simulink model "EZE557StEnCtrl"  (R2018b)
settings: Solver=FixedStepDiscrete  StartTime=0.0  StopTime=10.0  FixedStep=0.01  RelTol=1e-3
undefined symbols (not defined in the file or in its folder): data, KeSMSw4SSecRwLtStLgrstOtwdInwdClosePos1_Val, KeSMSw4SSecRwLtStLgrstUpwdDnwdClosePos1_Val, KeSMSw4SSecRwLtStLgrstUpwdDnwdClosePos2_Val, PassStBkReclnEn_Clear, PassStBkReclnEn_Set, PassStFwdBkwdEn_Clear, PassStFwdBkwdEn_Set, SecRwLtStBkReclnEn_Clear, SecRwLtStBkReclnEn_Set, SecRwLtStFwdBkwdEn_Clear, SecRwLtStFwdBkwdEn_Set, SecRwLtStLgrstInwdOtwdEn_Clear, SecRwLtStLgrstInwdOtwdEn_Set, SecRwLtStLgrstUpwdDnwdEn_Clear, SecRwLtStLgrstUpwdDnwdEn_Set, SecRwRtStBkReclnEn_Clear, SecRwRtStBkReclnEn_Set, SecRwRtStFwdBkwdEn_Clear, SecRwRtStFwdBkwdEn_Set, SecRwRtStLgrstInwdOtwdEn_Clear, SecRwRtStLgrstInwdOtwdEn_Set, SecRwRtStLgrstUpwdDnwdEn_Clear, SecRwRtStLgrstUpwdDnwdEn_Set, ThdRwLtStBkReclnEn_Clear, ThdRwLtStBkReclnEn_Set, ThdRwLtStCshnFldEn_Clear, ThdRwLtStCshnFldEn_Set, ThdRwLtStFwdBkwdEn_Clear, ThdRwLtStFwdBkwdEn_Set, ThdRwRtStBkReclnEn_Clear, ThdRwRtStBkReclnEn_Set, ThdRwRtStCshnFldEn_Clear, ThdRwRtStCshnFldEn_Set, ThdRwRtStFwdBkwdEn_Clear, ThdRwRtStFwdBkwdEn_Set, ZeroLEn_Clear, ZeroLEn_Set, ZeroREn_Clear, ZeroREn_Set
libraries: simulink x1
(part 1 of 2)
settings Model: Creator=sn2xws  LastModifiedBy=sn55gm
settings Model: ModifiedHistory=|
  | 2024.5.7 V1.0.0 557 eze模式
  | 2024.6.17 V1.1.0 座椅模式流程图V1.6
  | 2024.8.16 修复stage1会退出的问题
  | 2024.8.17 二排靠背电机目标位置异常问题修复
  | 2024.8.29 V3.0.3 V2.4流程，如果二排靠背小于目标位置，第一阶段不动二排靠背
  | 2024.9.25 V3.0.4 二排靠背reset条件改为只在第一阶段完成后reset一次
  | 2024.11.12 V3.0.5 第一阶段二排靠背到位置的flag替换
settings DataIOCC: SaveFormat=StructureWithTime
settings OptimizationCC: DefaultParameterBehavior=Inlined  EnhancedBackFolding=on  PassReuseOutputArgsAs=Individual arguments  ZeroExternalMemoryAtStartup=off  ZeroInternalMemoryAtStartup=off  OptimizeBlockOrder=speed  DifferentSizesBufferReuse=on  OptimizationCustomize=off
settings DebuggingCC: ParameterTunabilityLossMsg=error
settings SFSimCC: MATLABDynamicMemAlloc=off
settings RTWCC: SystemTargetFile=autosar.tlc  GenCodeOnly=on  TemplateMakefile=ert_default_tmf  Description=AUTOSAR  GenerateReport=on  IncludeHyperlinkInReport=on  LaunchReport=on  GenerateTraceInfo=on  GenerateTraceReport=on  GenerateTraceReportSl=on  GenerateTraceReportSf=on  GenerateTraceReportEml=on
settings CodeAppCC: ForceParamTrailComments=on  IgnoreCustomStorageClasses=off  OperatorAnnotations=on  SimulinkDataObjDesc=on  SFDataObjDesc=on  InsertBlockDesc=on
settings STFCustomTargetCC: TargetLangStandard=C99 (ISO)  MultiwordLength=256  ParMdlRefBuildCompliant=on  CompOptLevelCompliant=on  IncludeMdlTerminateFcn=off  CombineOutputUpdateFcns=on  SuppressErrorStatus=on  ERTCustomFileBanners=on  SupportNonFinite=off  SupportComplex=off  SupportContinuousTime=off  SupportNonInlinedSFcns=off  RemoveResetFunc=on  MATLABClassNameForMDSCustomization=Simulink.SoftwareTarget.ERTCustomization  AutosarCompliant=on  UseToolchainInfoCompliant=on  LookupTableObjectStructAxisOrder=2,1,3,4,...  LUTObjectStructOrderEvenSpacing=Size,Table,Breakpoints  SystemTargetFile=autosar.tlc
settings ERTTargetCC: TargetLangStandard=C99 (ISO)  ConcurrentExecutionCompliant=off  IncludeMdlTerminateFcn=off  SuppressErrorStatus=on  SupportNonFinite=off  SupportComplex=off  ModelStepFunctionPrototypeControlCompliant=off  CPPClassGenCompliant=off  AutosarCompliant=on  LookupTableObjectStructAxisOrder=2,1,3,4,...  LUTObjectStructOrderEvenSpacing=Size,Table,Breakpoints  InlinedParameterPlacement=NonHierarchical  ERTCustomFileTemplate=example_file_process.tlc  ERTFilePackagingFormat=Compact  BooleanTrueId=TRUE  BooleanFalseId=FALSE

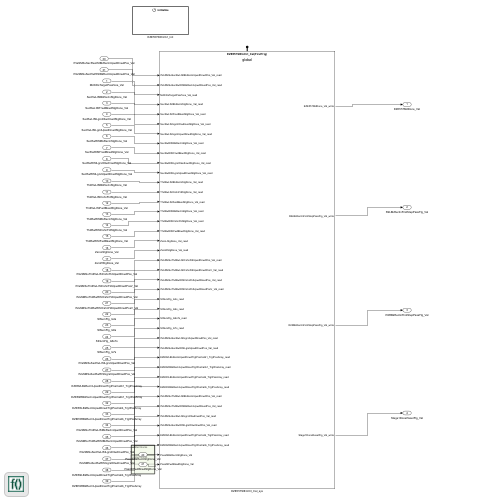
[thumbnail: Simulink's stored preview of the top-level diagram]
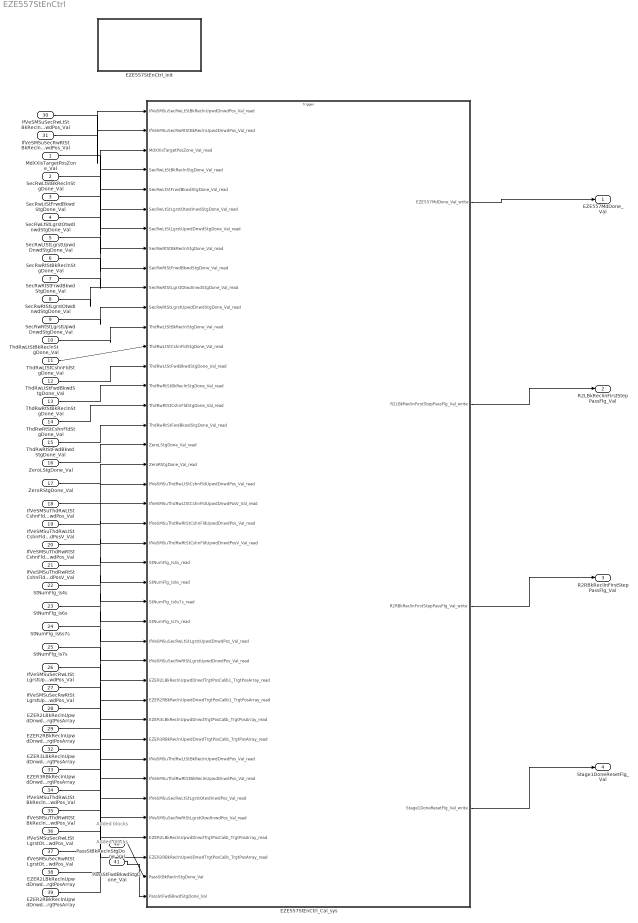
== system EZE557StEnCtrl ==
  note: Added blocks
  note: Added blocks
  MdXXIsTargetPosZone_Val : Inport  OutDataTypeStr=uint32  PortDimensions=1
  SecRwLtStBkReclnStgDone_Val : Inport  Port=2  OutDataTypeStr=boolean  PortDimensions=1
  SecRwLtStFrwdBkwdStgDone_Val : Inport  Port=3  OutDataTypeStr=boolean  PortDimensions=1
  SecRwLtStLgrstOtwdInwdStgDone_Val : Inport  Port=4  OutDataTypeStr=boolean  PortDimensions=1
  SecRwLtStLgrstUpwdDnwdStgDone_Val : Inport  Port=5  OutDataTypeStr=boolean  PortDimensions=1
  SecRwRtStBkReclnStgDone_Val : Inport  Port=6  OutDataTypeStr=boolean  PortDimensions=1
  SecRwRtStFrwdBkwdStgDone_Val : Inport  Port=7  OutDataTypeStr=boolean  PortDimensions=1
  SecRwRtStLgrstOtwdInwdStgDone_Val : Inport  Port=8  OutDataTypeStr=boolean  PortDimensions=1
  SecRwRtStLgrstUpwdDnwdStgDone_Val : Inport  Port=9  OutDataTypeStr=boolean  PortDimensions=1
  ThdRwLtStBkReclnStgDone_Val : Inport  Port=10  OutDataTypeStr=boolean  PortDimensions=1
  ThdRwLtStCshnFldStgDone_Val : Inport  Port=11  OutDataTypeStr=boolean  PortDimensions=1
  ThdRwLtStFwdBkwdStgDone_Val : Inport  Port=12  OutDataTypeStr=boolean  PortDimensions=1
  ThdRwRtStBkReclnStgDone_Val : Inport  Port=13  OutDataTypeStr=boolean  PortDimensions=1
  ThdRwRtStCshnFldStgDone_Val : Inport  Port=14  OutDataTypeStr=boolean  PortDimensions=1
  ThdRwRtStFwdBkwdStgDone_Val : Inport  Port=15  OutDataTypeStr=boolean  PortDimensions=1
  ZeroLStgDone_Val : Inport  Port=16  OutDataTypeStr=boolean  PortDimensions=1
  ZeroRStgDone_Val : Inport  Port=17  OutDataTypeStr=boolean  PortDimensions=1
  IfVeSMSuThdRwLtStCshnFldUpwdDnwdPos_Val : Inport  Port=18  OutDataTypeStr=uint16  PortDimensions=1
  IfVeSMSuThdRwLtStCshnFldUpwdDnwdPosV_Val : Inport  Port=19  OutDataTypeStr=boolean  PortDimensions=1
  IfVeSMSuThdRwRtStCshnFldUpwdDnwdPos_Val : Inport  Port=20  OutDataTypeStr=uint16  PortDimensions=1
  IfVeSMSuThdRwRtStCshnFldUpwdDnwdPosV_Val : Inport  Port=21  OutDataTypeStr=boolean  PortDimensions=1
  StNumFlg_Is4s : Inport  Port=22  OutDataTypeStr=boolean  PortDimensions=1
  StNumFlg_Is6s : Inport  Port=23  OutDataTypeStr=boolean  PortDimensions=1
  StNumFlg_Is6s7s : Inport  Port=24  OutDataTypeStr=boolean  PortDimensions=1
  StNumFlg_Is7s : Inport  Port=25  OutDataTypeStr=boolean  PortDimensions=1
  IfVeSMSuSecRwLtStLgrstUpwdDnwdPos_Val : Inport  Port=26  OutDataTypeStr=uint16  PortDimensions=1
  IfVeSMSuSecRwRtStLgrstUpwdDnwdPos_Val : Inport  Port=27  OutDataTypeStr=uint16  PortDimensions=1
  EZER2LBkReclnUpwdDnwdTrgtPosCalib1_TrgtPosArray : Inport  Description=|  Port=28  OutDataTypeStr=uint16  PortDimensions=3
      | 0:Pos
      | 1:Max
      | 2:Min
  EZER2RBkReclnUpwdDnwdTrgtPosCalib1_TrgtPosArray : Inport  Description=|  Port=29  OutDataTypeStr=uint16  PortDimensions=3
      | 0:Pos
      | 1:Max
      | 2:Min
  IfVeSMSuSecRwLtStBkReclnUpwdDnwdPos_Val : Inport  Port=30  OutDataTypeStr=uint16  PortDimensions=1
  IfVeSMSuSecRwRtStBkReclnUpwdDnwdPos_Val : Inport  Port=31  OutDataTypeStr=uint16  PortDimensions=1
  EZER3LBkReclnUpwdDnwdTrgtPosCalib_TrgtPosArray : Inport  Description=|  Port=32  OutDataTypeStr=uint16  PortDimensions=3
      | 0:Pos
      | 1:Max
      | 2:Min
  EZER3RBkReclnUpwdDnwdTrgtPosCalib_TrgtPosArray : Inport  Description=|  Port=33  OutDataTypeStr=uint16  PortDimensions=3
      | 0:Pos
      | 1:Max
      | 2:Min
  IfVeSMSuThdRwLtStBkReclnUpwdDnwdPos_Val : Inport  Port=34  OutDataTypeStr=uint16  PortDimensions=1
  IfVeSMSuThdRwRtStBkReclnUpwdDnwdPos_Val : Inport  Port=35  OutDataTypeStr=uint16  PortDimensions=1
  IfVeSMSuSecRwLtStLgrstOtwdInwdPos_Val : Inport  Port=36  OutDataTypeStr=uint16  PortDimensions=1
  IfVeSMSuSecRwRtStLgrstOtwdInwdPos_Val : Inport  Port=37  OutDataTypeStr=uint16  PortDimensions=1
  EZER2LBkReclnUpwdDnwdTrgtPosCalib_TrgtPosArray : Inport  Description=|  Port=38  OutDataTypeStr=uint16  PortDimensions=3
      | 0:Pos
      | 1:Max
      | 2:Min
  EZER2RBkReclnUpwdDnwdTrgtPosCalib_TrgtPosArray : Inport  Description=|  Port=39  OutDataTypeStr=uint16  PortDimensions=3
      | 0:Pos
      | 1:Max
      | 2:Min
  PassStBkReclnStgDone_Val : Inport  Port=40  OutDataTypeStr=boolean  PortDimensions=1
  PassStFwdBkwdStgDone_Val : Inport  Port=41  OutDataTypeStr=boolean  PortDimensions=1
  EZE557StEnCtrl_Cal_sys : Subsystem
  EZE557StEnCtrl_Init : Subsystem
  EZE557MdDone_Val : Outport  OutDataTypeStr=uint8  PortDimensions=1  VectorParamsAs1DForOutWhenUnconnected=off
  R2LBkReclinFirstStepPassFlg_Val : Outport  Port=2  OutDataTypeStr=boolean  PortDimensions=1  VectorParamsAs1DForOutWhenUnconnected=off
  R2RBkReclinFirstStepPassFlg_Val : Outport  Port=3  OutDataTypeStr=boolean  PortDimensions=1  VectorParamsAs1DForOutWhenUnconnected=off
  Stage1DoneResetFlg_Val : Outport  Port=4  OutDataTypeStr=boolean  PortDimensions=1  VectorParamsAs1DForOutWhenUnconnected=off
  wires:
  MdXXIsTargetPosZone_Val/1 -> EZE557StEnCtrl_Cal_sys/3(MdXXIsTargetPosZone_Val_read)
  SecRwLtStBkReclnStgDone_Val/1 -> EZE557StEnCtrl_Cal_sys/4(SecRwLtStBkReclnStgDone_Val_read)
  SecRwLtStFrwdBkwdStgDone_Val/1 -> EZE557StEnCtrl_Cal_sys/5(SecRwLtStFrwdBkwdStgDone_Val_read)
  SecRwLtStLgrstOtwdInwdStgDone_Val/1 -> EZE557StEnCtrl_Cal_sys/6(SecRwLtStLgrstOtwdInwdStgDone_Val_read)
  SecRwLtStLgrstUpwdDnwdStgDone_Val/1 -> EZE557StEnCtrl_Cal_sys/7(SecRwLtStLgrstUpwdDnwdStgDone_Val_read)
  SecRwRtStBkReclnStgDone_Val/1 -> EZE557StEnCtrl_Cal_sys/8(SecRwRtStBkReclnStgDone_Val_read)
  SecRwRtStFrwdBkwdStgDone_Val/1 -> EZE557StEnCtrl_Cal_sys/9(SecRwRtStFrwdBkwdStgDone_Val_read)
  SecRwRtStLgrstOtwdInwdStgDone_Val/1 -> EZE557StEnCtrl_Cal_sys/10(SecRwRtStLgrstOtwdInwdStgDone_Val_read)
  SecRwRtStLgrstUpwdDnwdStgDone_Val/1 -> EZE557StEnCtrl_Cal_sys/11(SecRwRtStLgrstUpwdDnwdStgDone_Val_read)
  ThdRwLtStBkReclnStgDone_Val/1 -> EZE557StEnCtrl_Cal_sys/12(ThdRwLtStBkReclnStgDone_Val_read)
  ThdRwLtStCshnFldStgDone_Val/1 -> EZE557StEnCtrl_Cal_sys/13(ThdRwLtStCshnFldStgDone_Val_read)
  ThdRwLtStFwdBkwdStgDone_Val/1 -> EZE557StEnCtrl_Cal_sys/14(ThdRwLtStFwdBkwdStgDone_Val_read)
  ThdRwRtStBkReclnStgDone_Val/1 -> EZE557StEnCtrl_Cal_sys/15(ThdRwRtStBkReclnStgDone_Val_read)
  ThdRwRtStCshnFldStgDone_Val/1 -> EZE557StEnCtrl_Cal_sys/16(ThdRwRtStCshnFldStgDone_Val_read)
  ThdRwRtStFwdBkwdStgDone_Val/1 -> EZE557StEnCtrl_Cal_sys/17(ThdRwRtStFwdBkwdStgDone_Val_read)
  ZeroLStgDone_Val/1 -> EZE557StEnCtrl_Cal_sys/18(ZeroLStgDone_Val_read)
  ZeroRStgDone_Val/1 -> EZE557StEnCtrl_Cal_sys/19(ZeroRStgDone_Val_read)
  EZE557StEnCtrl_Cal_sys/1(EZE557MdDone_Val_write) -> EZE557MdDone_Val/1
  IfVeSMSuThdRwLtStCshnFldUpwdDnwdPos_Val/1 -> EZE557StEnCtrl_Cal_sys/20(IfVeSMSuThdRwLtStCshnFldUpwdDnwdPos_Val_read)
  IfVeSMSuThdRwLtStCshnFldUpwdDnwdPosV_Val/1 -> EZE557StEnCtrl_Cal_sys/21(IfVeSMSuThdRwLtStCshnFldUpwdDnwdPosV_Val_read)
  IfVeSMSuThdRwRtStCshnFldUpwdDnwdPos_Val/1 -> EZE557StEnCtrl_Cal_sys/22(IfVeSMSuThdRwRtStCshnFldUpwdDnwdPos_Val_read)
  IfVeSMSuThdRwRtStCshnFldUpwdDnwdPosV_Val/1 -> EZE557StEnCtrl_Cal_sys/23(IfVeSMSuThdRwRtStCshnFldUpwdDnwdPosV_Val_read)
  StNumFlg_Is4s/1 -> EZE557StEnCtrl_Cal_sys/24(StNumFlg_Is4s_read)
  StNumFlg_Is6s/1 -> EZE557StEnCtrl_Cal_sys/25(StNumFlg_Is6s_read)
  StNumFlg_Is6s7s/1 -> EZE557StEnCtrl_Cal_sys/26(StNumFlg_Is6s7s_read)
  StNumFlg_Is7s/1 -> EZE557StEnCtrl_Cal_sys/27(StNumFlg_Is7s_read)
  IfVeSMSuSecRwLtStLgrstUpwdDnwdPos_Val/1 -> EZE557StEnCtrl_Cal_sys/28(IfVeSMSuSecRwLtStLgrstUpwdDnwdPos_Val_read)
  IfVeSMSuSecRwRtStLgrstUpwdDnwdPos_Val/1 -> EZE557StEnCtrl_Cal_sys/29(IfVeSMSuSecRwRtStLgrstUpwdDnwdPos_Val_read)
  EZER2LBkReclnUpwdDnwdTrgtPosCalib1_TrgtPosArray/1 -> EZE557StEnCtrl_Cal_sys/30(EZER2LBkReclnUpwdDnwdTrgtPosCalib1_TrgtPosArray_read)
  EZER2RBkReclnUpwdDnwdTrgtPosCalib1_TrgtPosArray/1 -> EZE557StEnCtrl_Cal_sys/31(EZER2RBkReclnUpwdDnwdTrgtPosCalib1_TrgtPosArray_read)
  IfVeSMSuSecRwLtStBkReclnUpwdDnwdPos_Val/1 -> EZE557StEnCtrl_Cal_sys/1(IfVeSMSuSecRwLtStBkReclnUpwdDnwdPos_Val_read)
  IfVeSMSuSecRwRtStBkReclnUpwdDnwdPos_Val/1 -> EZE557StEnCtrl_Cal_sys/2(IfVeSMSuSecRwRtStBkReclnUpwdDnwdPos_Val_read)
  EZE557StEnCtrl_Cal_sys/2(R2LBkReclinFirstStepPassFlg_Val_write) -> R2LBkReclinFirstStepPassFlg_Val/1
  EZE557StEnCtrl_Cal_sys/3(R2RBkReclinFirstStepPassFlg_Val_write) -> R2RBkReclinFirstStepPassFlg_Val/1
  EZER3LBkReclnUpwdDnwdTrgtPosCalib_TrgtPosArray/1 -> EZE557StEnCtrl_Cal_sys/32(EZER3LBkReclnUpwdDnwdTrgtPosCalib_TrgtPosArray_read)
  EZER3RBkReclnUpwdDnwdTrgtPosCalib_TrgtPosArray/1 -> EZE557StEnCtrl_Cal_sys/33(EZER3RBkReclnUpwdDnwdTrgtPosCalib_TrgtPosArray_read)
  IfVeSMSuThdRwLtStBkReclnUpwdDnwdPos_Val/1 -> EZE557StEnCtrl_Cal_sys/34(IfVeSMSuThdRwLtStBkReclnUpwdDnwdPos_Val_read)
  IfVeSMSuThdRwRtStBkReclnUpwdDnwdPos_Val/1 -> EZE557StEnCtrl_Cal_sys/35(IfVeSMSuThdRwRtStBkReclnUpwdDnwdPos_Val_read)
  EZE557StEnCtrl_Cal_sys/4(Stage1DoneResetFlg_Val_write) -> Stage1DoneResetFlg_Val/1
  IfVeSMSuSecRwLtStLgrstOtwdInwdPos_Val/1 -> EZE557StEnCtrl_Cal_sys/36(IfVeSMSuSecRwLtStLgrstOtwdInwdPos_Val_read)
  IfVeSMSuSecRwRtStLgrstOtwdInwdPos_Val/1 -> EZE557StEnCtrl_Cal_sys/37(IfVeSMSuSecRwRtStLgrstOtwdInwdPos_Val_read)
  EZER2LBkReclnUpwdDnwdTrgtPosCalib_TrgtPosArray/1 -> EZE557StEnCtrl_Cal_sys/38(EZER2LBkReclnUpwdDnwdTrgtPosCalib_TrgtPosArray_read)
  EZER2RBkReclnUpwdDnwdTrgtPosCalib_TrgtPosArray/1 -> EZE557StEnCtrl_Cal_sys/39(EZER2RBkReclnUpwdDnwdTrgtPosCalib_TrgtPosArray_read)
  PassStBkReclnStgDone_Val/1 -> EZE557StEnCtrl_Cal_sys/40(PassStBkReclnStgDone_Val)
  PassStFwdBkwdStgDone_Val/1 -> EZE557StEnCtrl_Cal_sys/41(PassStFwdBkwdStgDone_Val)

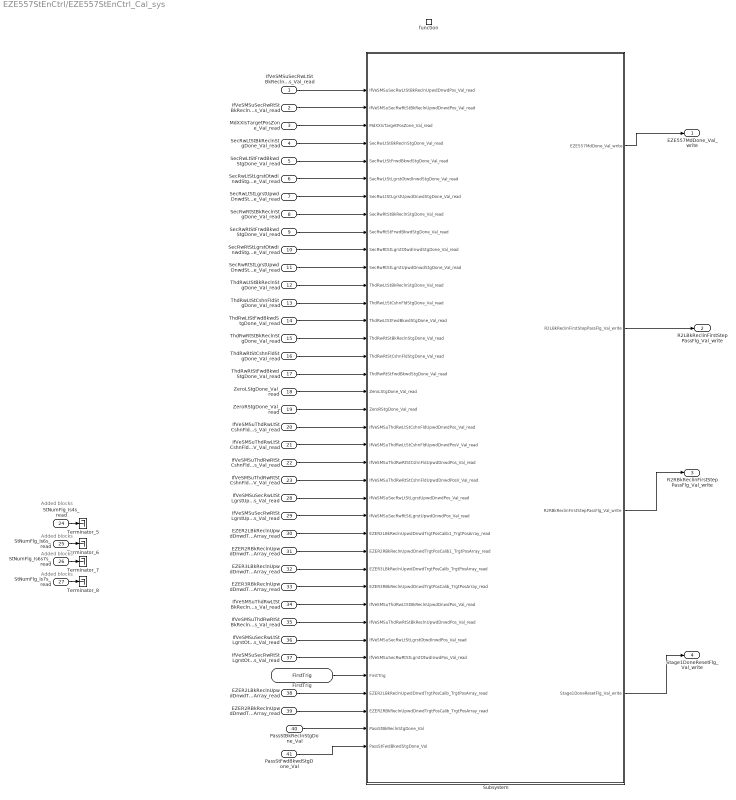
== system EZE557StEnCtrl/EZE557StEnCtrl_Cal_sys ==
  note: Added blocks
  note: Added blocks
  note: Added blocks
  note: Added blocks
  IfVeSMSuSecRwLtStBkReclnUpwdDnwdPos_Val_read : Inport
  IfVeSMSuSecRwRtStBkReclnUpwdDnwdPos_Val_read : Inport  Port=2
  MdXXIsTargetPosZone_Val_read : Inport  Port=3
  SecRwLtStBkReclnStgDone_Val_read : Inport  Port=4
  SecRwLtStFrwdBkwdStgDone_Val_read : Inport  Port=5
  SecRwLtStLgrstOtwdInwdStgDone_Val_read : Inport  Port=6
  SecRwLtStLgrstUpwdDnwdStgDone_Val_read : Inport  Port=7
  SecRwRtStBkReclnStgDone_Val_read : Inport  Port=8
  SecRwRtStFrwdBkwdStgDone_Val_read : Inport  Port=9
  SecRwRtStLgrstOtwdInwdStgDone_Val_read : Inport  Port=10
  SecRwRtStLgrstUpwdDnwdStgDone_Val_read : Inport  Port=11
  ThdRwLtStBkReclnStgDone_Val_read : Inport  Port=12
  ThdRwLtStCshnFldStgDone_Val_read : Inport  Port=13
  ThdRwLtStFwdBkwdStgDone_Val_read : Inport  Port=14
  ThdRwRtStBkReclnStgDone_Val_read : Inport  Port=15
  ThdRwRtStCshnFldStgDone_Val_read : Inport  Port=16
  ThdRwRtStFwdBkwdStgDone_Val_read : Inport  Port=17
  ZeroLStgDone_Val_read : Inport  Port=18
  ZeroRStgDone_Val_read : Inport  Port=19
  IfVeSMSuThdRwLtStCshnFldUpwdDnwdPos_Val_read : Inport  Port=20
  IfVeSMSuThdRwLtStCshnFldUpwdDnwdPosV_Val_read : Inport  Port=21
  IfVeSMSuThdRwRtStCshnFldUpwdDnwdPos_Val_read : Inport  Port=22
  IfVeSMSuThdRwRtStCshnFldUpwdDnwdPosV_Val_read : Inport  Port=23
  StNumFlg_Is4s_read : Inport  Port=24
  StNumFlg_Is6s_read : Inport  Port=25
  StNumFlg_Is6s7s_read : Inport  Port=26
  StNumFlg_Is7s_read : Inport  Port=27
  IfVeSMSuSecRwLtStLgrstUpwdDnwdPos_Val_read : Inport  Port=28
  IfVeSMSuSecRwRtStLgrstUpwdDnwdPos_Val_read : Inport  Port=29
  EZER2LBkReclnUpwdDnwdTrgtPosCalib1_TrgtPosArray_read : Inport  Port=30
  EZER2RBkReclnUpwdDnwdTrgtPosCalib1_TrgtPosArray_read : Inport  Port=31
  EZER3LBkReclnUpwdDnwdTrgtPosCalib_TrgtPosArray_read : Inport  Port=32
  EZER3RBkReclnUpwdDnwdTrgtPosCalib_TrgtPosArray_read : Inport  Port=33
  IfVeSMSuThdRwLtStBkReclnUpwdDnwdPos_Val_read : Inport  Port=34
  IfVeSMSuThdRwRtStBkReclnUpwdDnwdPos_Val_read : Inport  Port=35
  IfVeSMSuSecRwLtStLgrstOtwdInwdPos_Val_read : Inport  Port=36
  IfVeSMSuSecRwRtStLgrstOtwdInwdPos_Val_read : Inport  Port=37
  EZER2LBkReclnUpwdDnwdTrgtPosCalib_TrgtPosArray_read : Inport  Port=38
  EZER2RBkReclnUpwdDnwdTrgtPosCalib_TrgtPosArray_read : Inport  Port=39
  PassStBkReclnStgDone_Val : Inport  Port=40
  PassStFwdBkwdStgDone_Val : Inport  Port=41
  function : TriggerPort  TriggerType=function-call  IsSimulinkFunction=on  FunctionName=EZE557StEnCtrl_Cal  VariantControl=(inherit)
  Subsystem : Subsystem
  Terminator_{5..8} (4 alike) : Terminator
  FirstTrig : ArgIn  OutDataTypeStr=boolean  ArgumentName=FirstTrig
  EZE557MdDone_Val_write : Outport  VectorParamsAs1DForOutWhenUnconnected=off
      settings: EnsureOutportIsVirtual=on
  R2LBkReclinFirstStepPassFlg_Val_write : Outport  Port=2  VectorParamsAs1DForOutWhenUnconnected=off
      settings: EnsureOutportIsVirtual=on
  R2RBkReclinFirstStepPassFlg_Val_write : Outport  Port=3  VectorParamsAs1DForOutWhenUnconnected=off
      settings: EnsureOutportIsVirtual=on
  Stage1DoneResetFlg_Val_write : Outport  Port=4  VectorParamsAs1DForOutWhenUnconnected=off
      settings: EnsureOutportIsVirtual=on
  wires:
  MdXXIsTargetPosZone_Val_read/1 -> Subsystem/3(MdXXIsTargetPosZone_Val_read)
  SecRwLtStBkReclnStgDone_Val_read/1 -> Subsystem/4(SecRwLtStBkReclnStgDone_Val_read)
  SecRwLtStFrwdBkwdStgDone_Val_read/1 -> Subsystem/5(SecRwLtStFrwdBkwdStgDone_Val_read)
  SecRwLtStLgrstOtwdInwdStgDone_Val_read/1 -> Subsystem/6(SecRwLtStLgrstOtwdInwdStgDone_Val_read)
  SecRwLtStLgrstUpwdDnwdStgDone_Val_read/1 -> Subsystem/7(SecRwLtStLgrstUpwdDnwdStgDone_Val_read)
  SecRwRtStBkReclnStgDone_Val_read/1 -> Subsystem/8(SecRwRtStBkReclnStgDone_Val_read)
  SecRwRtStFrwdBkwdStgDone_Val_read/1 -> Subsystem/9(SecRwRtStFrwdBkwdStgDone_Val_read)
  SecRwRtStLgrstOtwdInwdStgDone_Val_read/1 -> Subsystem/10(SecRwRtStLgrstOtwdInwdStgDone_Val_read)
  SecRwRtStLgrstUpwdDnwdStgDone_Val_read/1 -> Subsystem/11(SecRwRtStLgrstUpwdDnwdStgDone_Val_read)
  ThdRwLtStBkReclnStgDone_Val_read/1 -> Subsystem/12(ThdRwLtStBkReclnStgDone_Val_read)
  ThdRwLtStCshnFldStgDone_Val_read/1 -> Subsystem/13(ThdRwLtStCshnFldStgDone_Val_read)
  ThdRwLtStFwdBkwdStgDone_Val_read/1 -> Subsystem/14(ThdRwLtStFwdBkwdStgDone_Val_read)
  ThdRwRtStBkReclnStgDone_Val_read/1 -> Subsystem/15(ThdRwRtStBkReclnStgDone_Val_read)
  ThdRwRtStCshnFldStgDone_Val_read/1 -> Subsystem/16(ThdRwRtStCshnFldStgDone_Val_read)
  ThdRwRtStFwdBkwdStgDone_Val_read/1 -> Subsystem/17(ThdRwRtStFwdBkwdStgDone_Val_read)
  ZeroLStgDone_Val_read/1 -> Subsystem/18(ZeroLStgDone_Val_read)
  ZeroRStgDone_Val_read/1 -> Subsystem/19(ZeroRStgDone_Val_read)
  Subsystem/1(EZE557MdDone_Val_write) -> EZE557MdDone_Val_write/1
  StNumFlg_Is4s_read/1 -> Terminator_5/1
  StNumFlg_Is6s_read/1 -> Terminator_6/1
  StNumFlg_Is6s7s_read/1 -> Terminator_7/1
  StNumFlg_Is7s_read/1 -> Terminator_8/1
  IfVeSMSuThdRwLtStCshnFldUpwdDnwdPos_Val_read/1 -> Subsystem/20(IfVeSMSuThdRwLtStCshnFldUpwdDnwdPos_Val_read)
  IfVeSMSuThdRwLtStCshnFldUpwdDnwdPosV_Val_read/1 -> Subsystem/21(IfVeSMSuThdRwLtStCshnFldUpwdDnwdPosV_Val_read)
  IfVeSMSuThdRwRtStCshnFldUpwdDnwdPos_Val_read/1 -> Subsystem/22(IfVeSMSuThdRwRtStCshnFldUpwdDnwdPos_Val_read)
  IfVeSMSuThdRwRtStCshnFldUpwdDnwdPosV_Val_read/1 -> Subsystem/23(IfVeSMSuThdRwRtStCshnFldUpwdDnwdPosV_Val_read)
  IfVeSMSuSecRwLtStLgrstUpwdDnwdPos_Val_read/1 -> Subsystem/24(IfVeSMSuSecRwLtStLgrstUpwdDnwdPos_Val_read)
  IfVeSMSuSecRwRtStLgrstUpwdDnwdPos_Val_read/1 -> Subsystem/25(IfVeSMSuSecRwRtStLgrstUpwdDnwdPos_Val_read)
  EZER2LBkReclnUpwdDnwdTrgtPosCalib1_TrgtPosArray_read/1 -> Subsystem/26(EZER2LBkReclnUpwdDnwdTrgtPosCalib1_TrgtPosArray_read)
  EZER2RBkReclnUpwdDnwdTrgtPosCalib1_TrgtPosArray_read/1 -> Subsystem/27(EZER2RBkReclnUpwdDnwdTrgtPosCalib1_TrgtPosArray_read)
  IfVeSMSuSecRwLtStBkReclnUpwdDnwdPos_Val_read/1 -> Subsystem/1(IfVeSMSuSecRwLtStBkReclnUpwdDnwdPos_Val_read)
  IfVeSMSuSecRwRtStBkReclnUpwdDnwdPos_Val_read/1 -> Subsystem/2(IfVeSMSuSecRwRtStBkReclnUpwdDnwdPos_Val_read)
  EZER3LBkReclnUpwdDnwdTrgtPosCalib_TrgtPosArray_read/1 -> Subsystem/28(EZER3LBkReclnUpwdDnwdTrgtPosCalib_TrgtPosArray_read)
  EZER3RBkReclnUpwdDnwdTrgtPosCalib_TrgtPosArray_read/1 -> Subsystem/29(EZER3RBkReclnUpwdDnwdTrgtPosCalib_TrgtPosArray_read)
  IfVeSMSuThdRwLtStBkReclnUpwdDnwdPos_Val_read/1 -> Subsystem/30(IfVeSMSuThdRwLtStBkReclnUpwdDnwdPos_Val_read)
  IfVeSMSuThdRwRtStBkReclnUpwdDnwdPos_Val_read/1 -> Subsystem/31(IfVeSMSuThdRwRtStBkReclnUpwdDnwdPos_Val_read)
  Subsystem/2(R2LBkReclinFirstStepPassFlg_Val_write) -> R2LBkReclinFirstStepPassFlg_Val_write/1
  Subsystem/3(R2RBkReclinFirstStepPassFlg_Val_write) -> R2RBkReclinFirstStepPassFlg_Val_write/1
  Subsystem/4(Stage1DoneResetFlg_Val_write) -> Stage1DoneResetFlg_Val_write/1
  IfVeSMSuSecRwLtStLgrstOtwdInwdPos_Val_read/1 -> Subsystem/32(IfVeSMSuSecRwLtStLgrstOtwdInwdPos_Val_read)
  IfVeSMSuSecRwRtStLgrstOtwdInwdPos_Val_read/1 -> Subsystem/33(IfVeSMSuSecRwRtStLgrstOtwdInwdPos_Val_read)
  FirstTrig/1 -> Subsystem/34(FirstTrig)
  EZER2LBkReclnUpwdDnwdTrgtPosCalib_TrgtPosArray_read/1 -> Subsystem/35(EZER2LBkReclnUpwdDnwdTrgtPosCalib_TrgtPosArray_read)
  EZER2RBkReclnUpwdDnwdTrgtPosCalib_TrgtPosArray_read/1 -> Subsystem/36(EZER2RBkReclnUpwdDnwdTrgtPosCalib_TrgtPosArray_read)
  PassStBkReclnStgDone_Val/1 -> Subsystem/37(PassStBkReclnStgDone_Val)
  PassStFwdBkwdStgDone_Val/1 -> Subsystem/38(PassStFwdBkwdStgDone_Val)

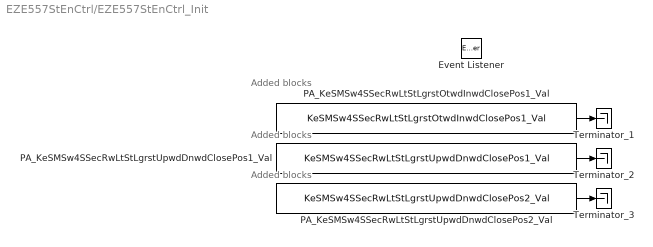
== system EZE557StEnCtrl/EZE557StEnCtrl_Init ==
  note: Added blocks
  note: Added blocks
  note: Added blocks
  Event Listener : EventListener  EventName=reset
  PA_KeSMSw4SSecRwLtStLgrstOtwdInwdClosePos1_Val : Constant  Value=KeSMSw4SSecRwLtStLgrstOtwdInwdClosePos1_Val
  PA_KeSMSw4SSecRwLtStLgrstUpwdDnwdClosePos1_Val : Constant  Value=KeSMSw4SSecRwLtStLgrstUpwdDnwdClosePos1_Val
  PA_KeSMSw4SSecRwLtStLgrstUpwdDnwdClosePos2_Val : Constant  Value=KeSMSw4SSecRwLtStLgrstUpwdDnwdClosePos2_Val
  Terminator_1 : Terminator
  Terminator_2 : Terminator
  Terminator_3 : Terminator
  wires:
  PA_KeSMSw4SSecRwLtStLgrstOtwdInwdClosePos1_Val/1 -> Terminator_1/1
  PA_KeSMSw4SSecRwLtStLgrstUpwdDnwdClosePos1_Val/1 -> Terminator_2/1
  PA_KeSMSw4SSecRwLtStLgrstUpwdDnwdClosePos2_Val/1 -> Terminator_3/1

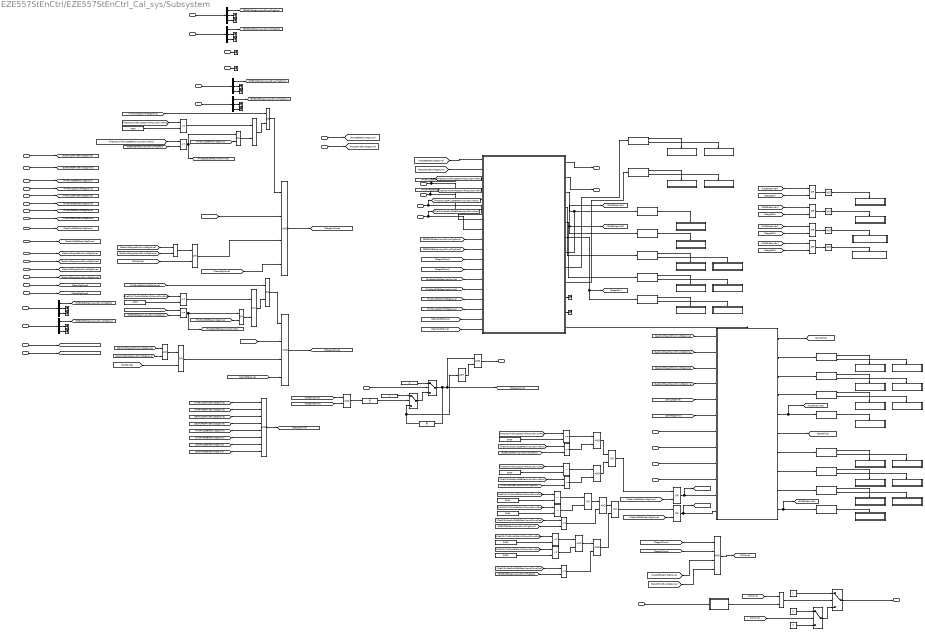
== system EZE557StEnCtrl/EZE557StEnCtrl_Cal_sys/Subsystem ==
  IfVeSMSuSecRwLtStBkReclnUpwdDnwdPos_Val_read : Inport
  IfVeSMSuSecRwRtStBkReclnUpwdDnwdPos_Val_read : Inport  Port=2
  MdXXIsTargetPosZone_Val_read : Inport  Port=3
  SecRwLtStBkReclnStgDone_Val_read : Inport  Port=4
  SecRwLtStFrwdBkwdStgDone_Val_read : Inport  Port=5
  SecRwLtStLgrstOtwdInwdStgDone_Val_read : Inport  Port=6
  SecRwLtStLgrstUpwdDnwdStgDone_Val_read : Inport  Port=7
  SecRwRtStBkReclnStgDone_Val_read : Inport  Port=8
  SecRwRtStFrwdBkwdStgDone_Val_read : Inport  Port=9
  SecRwRtStLgrstOtwdInwdStgDone_Val_read : Inport  Port=10
  SecRwRtStLgrstUpwdDnwdStgDone_Val_read : Inport  Port=11
  ThdRwLtStBkReclnStgDone_Val_read : Inport  Port=12
  ThdRwLtStCshnFldStgDone_Val_read : Inport  Port=13
  ThdRwLtStFwdBkwdStgDone_Val_read : Inport  Port=14
  ThdRwRtStBkReclnStgDone_Val_read : Inport  Port=15
  ThdRwRtStCshnFldStgDone_Val_read : Inport  Port=16
  ThdRwRtStFwdBkwdStgDone_Val_read : Inport  Port=17
  ZeroLStgDone_Val_read : Inport  Port=18
  ZeroRStgDone_Val_read : Inport  Port=19
  IfVeSMSuThdRwLtStCshnFldUpwdDnwdPos_Val_read : Inport  Port=20
  IfVeSMSuThdRwLtStCshnFldUpwdDnwdPosV_Val_read : Inport  Port=21
  IfVeSMSuThdRwRtStCshnFldUpwdDnwdPos_Val_read : Inport  Port=22
  IfVeSMSuThdRwRtStCshnFldUpwdDnwdPosV_Val_read : Inport  Port=23
  IfVeSMSuSecRwLtStLgrstUpwdDnwdPos_Val_read : Inport  Port=24
  IfVeSMSuSecRwRtStLgrstUpwdDnwdPos_Val_read : Inport  Port=25
  EZER2LBkReclnUpwdDnwdTrgtPosCalib1_TrgtPosArray_read : Inport  Port=26
  EZER2RBkReclnUpwdDnwdTrgtPosCalib1_TrgtPosArray_read : Inport  Port=27
  EZER3LBkReclnUpwdDnwdTrgtPosCalib_TrgtPosArray_read : Inport  Port=28
  EZER3RBkReclnUpwdDnwdTrgtPosCalib_TrgtPosArray_read : Inport  Port=29
  IfVeSMSuThdRwLtStBkReclnUpwdDnwdPos_Val_read : Inport  Port=30
  IfVeSMSuThdRwRtStBkReclnUpwdDnwdPos_Val_read : Inport  Port=31
  IfVeSMSuSecRwLtStLgrstOtwdInwdPos_Val_read : Inport  Port=32
  IfVeSMSuSecRwRtStLgrstOtwdInwdPos_Val_read : Inport  Port=33
  FirstTrig : Inport  Port=34
  EZER2LBkReclnUpwdDnwdTrgtPosCalib_TrgtPosArray_read : Inport  Port=35
  EZER2RBkReclnUpwdDnwdTrgtPosCalib_TrgtPosArray_read : Inport  Port=36
  PassStBkReclnStgDone_Val : Inport  Port=37
  PassStFwdBkwdStgDone_Val : Inport  Port=38
  32BitSelector : Subsystem  mask(32 Bit Selector){BitNum=0}
      mask prompts: BitNum "Select Bit Number"
      mask help: Allows selection of a particular bit (0-31) out of a packed word up to 32 bits long. Output will be true if the bit number selected via the mask parameter is equal to one.
      mask TypeOptions BitNum: 0 | 1 | 2 | 3 | 4 | 5 | 6 | 7 | 8 | 9 | 10 | 11 | 12 | 13 | 14 | 15 | 16 | 17 | 18 | 19 | 20 | 21 | 22 | 23 | 24 | 25 | 26 | 27 | 28 | 29 | 30 | 31
      mask Display:
      | text(0.5, 0.8,'BIT','horizontalAlignment','center')
      | text(0.5, 0.5,'SELECTOR','horizontalAlignment','center')
      | text(0.5, 0.2,['-- Bit ',char(get_param(gcb,'BitNum')),' --'],'horizontalAlignment','center')
  Chart : Stateflow chart  TreatAsAtomicUnit=on
  Constant : Constant  OutDataTypeStr=uint8
  Constant1 : Constant  Value=2  OutDataTypeStr=uint8
  Constant{7..9,11..13} (6 alike) : Constant  Value=3960  OutDataTypeStr=uint16  SampleTime=-1
  Constant2 : Constant  Value=0  OutDataTypeStr=uint8
  Constant3 : Constant  Value=4000  OutDataTypeStr=uint16  SampleTime=-1
  Constant4 : Constant  Value=4000  OutDataTypeStr=uint16  SampleTime=-1
  Constant5 : Constant  Value=0
  Constant6 : Constant
  Demux{,1..5} (6 alike) : Demux  Outputs=3
  If Action Subsystem1 : Subsystem  TreatAsAtomicUnit=on
  If Action Subsystem10 : Subsystem  TreatAsAtomicUnit=on
  If Action Subsystem11 : Subsystem  TreatAsAtomicUnit=on
  If Action Subsystem12 : Subsystem  TreatAsAtomicUnit=on
  If Action Subsystem13 : Subsystem  TreatAsAtomicUnit=on
  If Action Subsystem14 : Subsystem  TreatAsAtomicUnit=on
  If Action Subsystem15 : Subsystem  TreatAsAtomicUnit=on
  If Action Subsystem16 : Subsystem  TreatAsAtomicUnit=on
  If Action Subsystem17 : Subsystem  TreatAsAtomicUnit=on
  If Action Subsystem18 : Subsystem  TreatAsAtomicUnit=on
  If Action Subsystem19 : Subsystem  TreatAsAtomicUnit=on
  If Action Subsystem2 : Subsystem  TreatAsAtomicUnit=on
  If Action Subsystem20 : Subsystem  TreatAsAtomicUnit=on
  If Action Subsystem21 : Subsystem  TreatAsAtomicUnit=on
  If Action Subsystem22 : Subsystem  TreatAsAtomicUnit=on
  If Action Subsystem23 : Subsystem  TreatAsAtomicUnit=on
  If Action Subsystem24 : Subsystem  TreatAsAtomicUnit=on
  If Action Subsystem25 : Subsystem  TreatAsAtomicUnit=on
  If Action Subsystem26 : Subsystem  TreatAsAtomicUnit=on
  If Action Subsystem27 : Subsystem  TreatAsAtomicUnit=on
  If Action Subsystem28 : Subsystem  TreatAsAtomicUnit=on
  If Action Subsystem3 : Subsystem  TreatAsAtomicUnit=on
  If Action Subsystem4 : Subsystem  TreatAsAtomicUnit=on
  If Action Subsystem5 : Subsystem  TreatAsAtomicUnit=on
  If Action Subsystem6 : Subsystem  TreatAsAtomicUnit=on
  If Action Subsystem7 : Subsystem  TreatAsAtomicUnit=on
  If Action Subsystem8 : Subsystem  TreatAsAtomicUnit=on
  If Action Subsystem9 : Subsystem  TreatAsAtomicUnit=on
  If{1,6,14..15} (4 alike) : If  IfExpression=u1  ShowElse=off
  If{2..5,7..13} (11 alike) : If  IfExpression=u1
  Logical Operator : Logic  Inputs=4  AllPortsSameDT=off  OutDataTypeStr=boolean
  Logical Operator{1..2,10,12,14,16,19,21..25,29,33..34} (15 alike) : Logic  Operator=OR  AllPortsSameDT=off  OutDataTypeStr=boolean
  Logical Operator{11,13,15,17,27} (5 alike) : Logic  Operator=NOT  AllPortsSameDT=off  OutDataTypeStr=boolean
  Logical Operator{4,6,8..9,18,20,26,28,30,32,35..36} (12 alike) : Logic  AllPortsSameDT=off  OutDataTypeStr=boolean
  Logical Operator3 : Logic  Inputs=4  AllPortsSameDT=off  OutDataTypeStr=boolean
  Logical Operator5 : Logic  Inputs=4  AllPortsSameDT=off  OutDataTypeStr=boolean
  Logical Operator7 : Logic  Inputs=8  AllPortsSameDT=off  OutDataTypeStr=boolean
  Relational Operator{,1,4,11,13,15} (6 alike) : RelationalOperator  Operator=<=  OutDataTypeStr=boolean  RndMeth=Simplest
  Relational Operator10 : RelationalOperator  Operator=<  OutDataTypeStr=boolean  RndMeth=Simplest
  Relational Operator{2..3,14,16..17} (5 alike) : RelationalOperator  OutDataTypeStr=boolean  RndMeth=Simplest
  Relational Operator8 : RelationalOperator  Operator=<  OutDataTypeStr=boolean  RndMeth=Simplest
  Relational Operator9 : RelationalOperator  Operator=<  OutDataTypeStr=boolean  RndMeth=Simplest
  Subsystem : Subsystem
  Subsystem1 : Subsystem
  Subsystem2 : Subsystem
  Switch{,1..3} (4 alike) : Switch  Criteria=u2 > Threshold
  Terminator_{1..16} (16 alike) : Terminator
  Unit Delay1 : UnitDelay  SampleTime=-1  HasFrameUpgradeWarning=on
  Unit Delay2 : UnitDelay  SampleTime=-1  HasFrameUpgradeWarning=on
  EZE557MdDone_Val_write : Outport  VectorParamsAs1DForOutWhenUnconnected=off
      settings: EnsureOutportIsVirtual=on
  R2LBkReclinFirstStepPassFlg_Val_write : Outport  Port=2  VectorParamsAs1DForOutWhenUnconnected=off
      settings: EnsureOutportIsVirtual=on
  R2RBkReclinFirstStepPassFlg_Val_write : Outport  Port=3  VectorParamsAs1DForOutWhenUnconnected=off
      settings: EnsureOutportIsVirtual=on
  Stage1DoneResetFlg_Val_write : Outport  Port=4  VectorParamsAs1DForOutWhenUnconnected=off
      settings: EnsureOutportIsVirtual=on
  wires:
  SecRwRtStBkReclnStgDone_Val_read/1 -> [SecRwRtStBkReclnStgDone]
  SecRwRtStFrwdBkwdStgDone_Val_read/1 -> [SecRwRtStFrwdBkwdStgDone]
  SecRwLtStFrwdBkwdStgDone_Val_read/1 -> [SecRwLtStFrwdBkwdStgDone]
  SecRwLtStBkReclnStgDone_Val_read/1 -> [SecRwLtStBkReclnStgDone]
  ThdRwLtStBkReclnStgDone_Val_read/1 -> [ThdRwLtStBkReclnStgDone]
  ThdRwLtStCshnFldStgDone_Val_read/1 -> [ThdRwLtStCshnFldStgDone]
  ThdRwLtStFwdBkwdStgDone_Val_read/1 -> [ThdRwLtStFwdBkwdStgDone]
  ThdRwRtStBkReclnStgDone_Val_read/1 -> [ThdRwRtStBkReclnStgDone]
  ThdRwRtStCshnFldStgDone_Val_read/1 -> [ThdRwRtStCshnFldStgDone]
  ThdRwRtStFwdBkwdStgDone_Val_read/1 -> [ThdRwRtStFwdBkwdStgDone]
  [ThdRwLtStBkReclnStgDone] -> Chart/3(ThdRwLtStBkReclnStgDone)
  [ThdRwRtStBkReclnStgDone] -> Chart/4(ThdRwRtStBkReclnStgDone)
  IfVeSMSuSecRwLtStLgrstUpwdDnwdPos_Val_read/1 -> Subsystem/7(IfVeSMSuSecRwLtStLgrstUpwdDnwdPos_Val_read)
  IfVeSMSuSecRwRtStLgrstUpwdDnwdPos_Val_read/1 -> Subsystem/8(IfVeSMSuSecRwRtStLgrstUpwdDnwdPos_Val_read)
  Chart/12(TrigComfortMd()) -> Subsystem/Trigger
  IfVeSMSuThdRwLtStCshnFldUpwdDnwdPos_Val_read/1 -> [IfVeSMSuThdRwLtStCshnFldUpwdDnwdPos], Chart/5(IfVeSMSuThdRwLtStCshnFldUpwdDnwdPos)
  IfVeSMSuThdRwRtStCshnFldUpwdDnwdPos_Val_read/1 -> Chart/6(IfVeSMSuThdRwRtStCshnFldUpwdDnwdPos), [IfVeSMSuThdRwRtStCshnFldUpwdDnwdPos]
  IfVeSMSuThdRwLtStCshnFldUpwdDnwdPosV_Val_read/1 -> Terminator_9/1
  IfVeSMSuThdRwRtStCshnFldUpwdDnwdPosV_Val_read/1 -> Terminator_10/1
  IfVeSMSuSecRwLtStBkReclnUpwdDnwdPos_Val_read/1 -> [IfVeSMSuSecRwLtStBkReclnUpwdDnwdPos], Chart/7(IfVeSMSuSecRwLtStBkReclnUpwdDnwdPos)
  IfVeSMSuSecRwRtStBkReclnUpwdDnwdPos_Val_read/1 -> Chart/8(IfVeSMSuSecRwRtStBkReclnUpwdDnwdPos), [IfVeSMSuSecRwRtStBkReclnUpwdDnwdPos]
  EZER2RBkReclnUpwdDnwdTrgtPosCalib1_TrgtPosArray_read/1 -> Demux1/1
  EZER2LBkReclnUpwdDnwdTrgtPosCalib1_TrgtPosArray_read/1 -> Demux/1
  Demux/1 -> [EZER2LBkReclnUpwdDnwdTrgtPos1]
  Demux1/1 -> [EZER2RBkReclnUpwdDnwdTrgtPos1]
  Demux/2 -> Terminator_1/1
  Demux/3 -> Terminator_2/1
  Demux1/2 -> Terminator_3/1
  Demux1/3 -> Terminator_4/1
  [EZER2LBkReclnUpwdDnwdTrgtPos1] -> Chart/9(EZER2LBkReclnUpwdDnwdTrgtPos1)
  [EZER2RBkReclnUpwdDnwdTrgtPos1] -> Chart/10(EZER2RBkReclnUpwdDnwdTrgtPos1)
  Chart/1(R2LBkReclinFirstStepPassFlg) -> R2LBkReclinFirstStepPassFlg_Val_write/1
  Chart/2(R2RBkReclinFirstStepPassFlg) -> R2RBkReclinFirstStepPassFlg_Val_write/1
  Logical Operator/1 -> [Stage1LDone]
  SecRwLtStLgrstOtwdInwdStgDone_Val_read/1 -> [SecRwLtStLgrstOtwdInwdStgDone]
  SecRwRtStLgrstOtwdInwdStgDone_Val_read/1 -> [SecRwRtStLgrstOtwdInwdStgDone]
  SecRwLtStLgrstUpwdDnwdStgDone_Val_read/1 -> [SecRwLtStLgrstUpwdDnwdStgDone]
  SecRwRtStLgrstUpwdDnwdStgDone_Val_read/1 -> [SecRwRtStLgrstUpwdDnwdStgDone]
  ZeroLStgDone_Val_read/1 -> [ZeroLStgDone]
  ZeroRStgDone_Val_read/1 -> [ZeroRStgDone]
  [SecRwLtStLgrstOtwdInwdStgDone] -> Subsystem/1(SecRwLtStLgrstOtwdInwdStgDone_Val_read)
  [SecRwLtStLgrstUpwdDnwdStgDone] -> Subsystem/2(SecRwLtStLgrstUpwdDnwdStgDone_Val_read)
  [SecRwRtStLgrstOtwdInwdStgDone] -> Subsystem/3(SecRwRtStLgrstOtwdInwdStgDone_Val_read)
  [SecRwRtStLgrstUpwdDnwdStgDone] -> Subsystem/4(SecRwRtStLgrstUpwdDnwdStgDone_Val_read)
  [ZeroLStgDone] -> Subsystem/5(ZeroLStgDone_Val_read)
  [ZeroRStgDone] -> Subsystem/6(ZeroRStgDone_Val_read)
  [ZeroLStgDone] -> Logical Operator/4
  Logical Operator2/1 -> Logical Operator3/1
  [ZeroRStgDone] -> Logical Operator3/4
  Logical Operator3/1 -> [Stage1RDone]
  [Stage1LDone] -> Logical Operator4/1
  [Stage1RDone] -> Logical Operator4/2
  Logical Operator4/1 -> Unit Delay1/1
  [Stage1Done] -> Chart/11(Stage1Done)
  [Stage2Done] -> Logical Operator5/2
  [Stage2Done] -> Chart/12(Stage2Done)
  Logical Operator7/1 -> [Stage2Done]
  [ThdRwLtStFwdBkwdStgDone] -> Logical Operator7/1
  [ThdRwRtStFwdBkwdStgDone] -> Logical Operator7/2
  [SecRwRtStFrwdBkwdStgDone] -> Logical Operator7/4
  [SecRwLtStFrwdBkwdStgDone] -> Logical Operator7/3
  [ThdRwLtStBkReclnStgDone] -> Logical Operator7/5
  [ThdRwRtStBkReclnStgDone] -> Logical Operator7/6
  Logical Operator5/1 -> [AllDone]
  Relational Operator/1 -> Logical Operator23/1, [FirstStgR3RBkReclnNotMovFlg]
  IfVeSMSuThdRwRtStBkReclnUpwdDnwdPos_Val_read/1 -> [IfVeSMSuThdRwRtStBkReclnUpwdDnwdPos]
  IfVeSMSuThdRwLtStBkReclnUpwdDnwdPos_Val_read/1 -> [IfVeSMSuThdRwLtStBkReclnUpwdDnwdPos]
  EZER3LBkReclnUpwdDnwdTrgtPosCalib_TrgtPosArray_read/1 -> Demux2/1
  Demux2/2 -> Terminator_5/1
  Demux2/3 -> Terminator_6/1
  Demux2/1 -> [EZER3LBkReclnUpwdDnwdTrgtPos]
  Demux3/1 -> [EZER3RBkReclnUpwdDnwdTrgtPos]
  Demux3/3 -> Terminator_12/1
  Demux3/2 -> Terminator_7/1
  EZER3RBkReclnUpwdDnwdTrgtPosCalib_TrgtPosArray_read/1 -> Demux3/1
  [IfVeSMSuThdRwRtStBkReclnUpwdDnwdPos] -> Relational Operator/1
  [EZER3RBkReclnUpwdDnwdTrgtPos] -> Relational Operator/2
  Relational Operator1/1 -> [FirstStgR3LBkReclnNotMovFlg], Logical Operator1/1
  [IfVeSMSuThdRwLtStBkReclnUpwdDnwdPos] -> Relational Operator1/1
  [EZER3LBkReclnUpwdDnwdTrgtPos] -> Relational Operator1/2
  [FirstStgR3LBkReclnNotMovFlg] -> Chart/13(FirstStgR3LBkReclnNotMovFlg)
  [FirstStgR3RBkReclnNotMovFlg] -> Chart/14(FirstStgR3RBkReclnNotMovFlg)
  [Stage1Done] -> Logical Operator5/1
  [AllDone] -> Switch1/2
  Constant/1 -> Switch/1
  Switch1/1 -> Switch/3
  32BitSelector/1(y) -> Logical Operator9/2
  Constant1/1 -> Switch1/1
  Constant2/1 -> Switch1/3
  [AllDone] -> Logical Operator9/1
  Logical Operator9/1 -> Switch/2
  Switch/1 -> EZE557MdDone_Val_write/1
  MdXXIsTargetPosZone_Val_read/1 -> 32BitSelector/1(x)
  If6/1 -> If Action Subsystem12/Action
  Chart/7(R3LBkReclnEn) -> [R3LBkReclinEn], If6/1
  Chart/3(R3RBkReclnEn) -> If1/1, [R3RBkReclinEn]
  If1/1 -> If Action Subsystem1/Action
  If2/1 -> If Action Subsystem3/Action
  If2/2 -> If Action Subsystem4/Action
  Chart/4(R3LCshnFldEn) -> If2/1
  Chart/5(R3RCshnFldEn) -> If3/1
  If3/2 -> If Action Subsystem6/Action
  If3/1 -> If Action Subsystem5/Action
  If7/1 -> If Action Subsystem9/Action
  If7/2 -> If Action Subsystem10/Action
  Chart/6(Stage2En) -> If7/1, [Stage2En]
  If8/2 -> If Action Subsystem11/Action
  If8/1 -> If Action Subsystem14/Action
  Subsystem/2(R2LLgrstInwdOtwdEn) -> If8/1
  Subsystem/3(R2LLgrstUpwdDnwdEn) -> If9/1
  If9/1 -> If Action Subsystem16/Action
  If9/2 -> If Action Subsystem15/Action
  If10/2 -> If Action Subsystem17/Action
  If10/1 -> If Action Subsystem18/Action
  Subsystem/4(R2LZeroEn) -> If10/1
  Subsystem/7(R2RLgrstInwdOtwdEn) -> If11/1
  If11/1 -> If Action Subsystem20/Action
  If11/2 -> If Action Subsystem19/Action
  If12/2 -> If Action Subsystem21/Action
  If12/1 -> If Action Subsystem22/Action
  Subsystem/8(R2RLgrstUpwdDnwdEn) -> If12/1
  Subsystem/9(R2RZeroEn) -> If13/1
  If13/1 -> If Action Subsystem24/Action
  If13/2 -> If Action Subsystem23/Action
  Logical Operator10/1 -> Logical Operator11/1
  Logical Operator13/1 -> If Action Subsystem2/Enable
  Logical Operator12/1 -> Logical Operator13/1
  [Stage2En] -> Logical Operator12/2
  [R3RBkReclinEn] -> Logical Operator12/1
  [R2LBkReclinEn] -> Logical Operator14/1
  [Stage2En] -> Logical Operator14/2
  Logical Operator14/1 -> Logical Operator15/1
  Logical Operator15/1 -> Subsystem1/Enable
  Logical Operator17/1 -> Subsystem2/Enable
  Logical Operator16/1 -> Logical Operator17/1
  [Stage2En] -> Logical Operator16/2
  [R2RBkReclinEn] -> Logical Operator16/1
  Subsystem/6(R2RFailflg) -> [R2RFailflg]
  [ThdRwRtStCshnFldStgDone] -> Chart/15(ThdRwRtStCshnFldStgDone)
  [ThdRwLtStCshnFldStgDone] -> Chart/16(ThdRwLtStCshnFldStgDone)
  Subsystem/1(R2LFailflg) -> [R2LFailflg]
  [SecRwLtStLgrstOtwdInwdStgDone] -> Logical Operator18/1
  [SecRwLtStLgrstUpwdDnwdStgDone] -> Logical Operator18/2
  Logical Operator18/1 -> Logical Operator19/1
  [R2LFailflg] -> Logical Operator19/2
  Logical Operator19/1 -> Logical Operator/3
  [SecRwRtStLgrstOtwdInwdStgDone] -> Logical Operator20/1
  [SecRwRtStLgrstUpwdDnwdStgDone] -> Logical Operator20/2
  Logical Operator20/1 -> Logical Operator21/1
  [R2RFailflg] -> Logical Operator21/2
  Logical Operator21/1 -> Logical Operator3/3
  [IfVeSMSuThdRwLtStCshnFldUpwdDnwdPos] -> Relational Operator2/1
  Constant3/1 -> Relational Operator2/2
  Relational Operator2/1 -> Logical Operator8/1
  Logical Operator1/1 -> Logical Operator8/2
  [ThdRwLtStBkReclnStgDone] -> Logical Operator1/2
  Logical Operator8/1 -> Logical Operator22/2
  [ThdRwLtStCshnFldStgDone] -> Logical Operator22/1
  Logical Operator22/1 -> Logical Operator/1
  Logical Operator6/1 -> Logical Operator2/2
  [ThdRwRtStCshnFldStgDone] -> Logical Operator2/1
  [IfVeSMSuThdRwRtStCshnFldUpwdDnwdPos] -> Relational Operator3/1
  Constant4/1 -> Relational Operator3/2
  Relational Operator3/1 -> Logical Operator6/1
  Logical Operator23/1 -> Logical Operator6/2
  [ThdRwRtStBkReclnStgDone] -> Logical Operator23/2
  IfVeSMSuSecRwLtStLgrstOtwdInwdPos_Val_read/1 -> Subsystem/9(IfVeSMSuSecRwLtStLgrstOtwdInwdPos_Val_read)
  IfVeSMSuSecRwRtStLgrstOtwdInwdPos_Val_read/1 -> Subsystem/10(IfVeSMSuSecRwRtStLgrstOtwdInwdPos_Val_read)
  If14/1 -> If Action Subsystem25/Action
  Subsystem/5(R2LBkReclnEn) -> [R2LBkReclinEn], If14/1
  If15/1 -> If Action Subsystem26/Action
  Subsystem/10(R2RBkReclnEn) -> [R2RBkReclinEn], If15/1
  [R3LBkReclinEn] -> Logical Operator10/1
  [Stage2En] -> Logical Operator10/2
  Logical Operator11/1 -> If Action Subsystem13/Enable
  FirstTrig/1 -> Switch2/2
  Constant5/1 -> Switch2/1
  Switch2/1 -> Logical Operator26/1, [Stage1Done], Unit Delay2/1
  Unit Delay1/1 -> Switch3/2
  Constant6/1 -> Switch3/1
  Switch3/1 -> Switch2/3
  Unit Delay2/1 -> Logical Operator27/1, Switch3/3
  [SecRwLtStBkReclnStgDone] -> Logical Operator7/7
  [SecRwRtStBkReclnStgDone] -> Logical Operator7/8
  [IfVeSMSuSecRwLtStBkReclnUpwdDnwdPos] -> Relational Operator4/1
  [EZER2LBkReclnUpwdDnwdTrgtPos1] -> Relational Operator4/2
  Logical Operator24/1 -> [Stg1R2LBkDone], Subsystem/11(SecRwLtStBkReclnStgDone)
  [SecRwLtStBkReclnStgDone] -> Logical Operator24/2
  Logical Operator25/1 -> [Stg1R2RBkDone], Subsystem/12(SecRwRtStBkReclnStgDone)
  [SecRwRtStBkReclnStgDone] -> Logical Operator25/2
  [Stg1R2LBkDone] -> Logical Operator/2
  [Stg1R2RBkDone] -> Logical Operator3/2
  Relational Operator8/1 -> Logical Operator28/1
  Constant7/1 -> Relational Operator8/2
  [IfVeSMSuThdRwLtStCshnFldUpwdDnwdPos] -> Relational Operator8/1
  Relational Operator4/1 -> Logical Operator28/2
  [IfVeSMSuThdRwLtStCshnFldUpwdDnwdPos] -> Relational Operator9/1
  Constant8/1 -> Relational Operator9/2
  Relational Operator9/1 -> Logical Operator29/1
  Relational Operator10/1 -> Logical Operator29/2
  Constant9/1 -> Relational Operator10/2
  [IfVeSMSuThdRwRtStCshnFldUpwdDnwdPos] -> Relational Operator10/1
  Logical Operator29/1 -> Logical Operator30/1
  Relational Operator11/1 -> Logical Operator30/2
  [EZER2RBkReclnUpwdDnwdTrgtPos1] -> Relational Operator11/2
  [IfVeSMSuSecRwRtStBkReclnUpwdDnwdPos] -> Relational Operator11/1
  Demux4/3 -> Terminator_11/1
  Demux4/2 -> Terminator_8/1
  Demux4/1 -> [EZER2LBkReclnUpwdDnwdTrgtPos]
  EZER2LBkReclnUpwdDnwdTrgtPosCalib_TrgtPosArray_read/1 -> Demux4/1
  Demux5/1 -> [EZER2RBkReclnUpwdDnwdTrgtPos]
  Demux5/2 -> Terminator_14/1
  Demux5/3 -> Terminator_13/1
  EZER2RBkReclnUpwdDnwdTrgtPosCalib_TrgtPosArray_read/1 -> Demux5/1
  Relational Operator13/1 -> Logical Operator32/2
  [IfVeSMSuThdRwLtStCshnFldUpwdDnwdPos] -> Relational Operator14/1
  Constant11/1 -> Relational Operator14/2
  Relational Operator14/1 -> Logical Operator32/1
  [EZER2LBkReclnUpwdDnwdTrgtPos] -> Relational Operator13/2
  [IfVeSMSuSecRwLtStBkReclnUpwdDnwdPos] -> Relational Operator13/1
  Logical Operator33/1 -> Logical Operator24/1
  Logical Operator32/1 -> Logical Operator33/1
  Logical Operator28/1 -> Logical Operator33/2
  Logical Operator30/1 -> Logical Operator34/1
  Logical Operator34/1 -> Logical Operator25/1
  [IfVeSMSuSecRwRtStBkReclnUpwdDnwdPos] -> Relational Operator15/1
  [EZER2RBkReclnUpwdDnwdTrgtPos] -> Relational Operator15/2
  [IfVeSMSuThdRwRtStCshnFldUpwdDnwdPos] -> Relational Operator16/1
  Relational Operator16/1 -> Logical Operator35/2
  Relational Operator17/1 -> Logical Operator35/1
  Constant12/1 -> Relational Operator17/2
  [IfVeSMSuThdRwLtStCshnFldUpwdDnwdPos] -> Relational Operator17/1
  Logical Operator35/1 -> Logical Operator36/1
  Relational Operator15/1 -> Logical Operator36/2
  Logical Operator36/1 -> Logical Operator34/2
  Constant13/1 -> Relational Operator16/2
  Logical Operator26/1 -> Stage1DoneResetFlg_Val_write/1
  Logical Operator27/1 -> Logical Operator26/2
  [Stg1R2RBkDone] -> Chart/17(SecRwRtStBkReclnStgDone)
  [Stg1R2LBkDone] -> Chart/18(SecRwLtStBkReclnStgDone)
  PassStBkReclnStgDone_Val/1 -> [PassStBkReclnStgDone]
  PassStFwdBkwdStgDone_Val/1 -> [PassStFwdBkwdStgDone]
  [PassStFwdBkwdStgDone] -> Chart/2(PassStFwdBkwdStgDone)
  [PassStBkReclnStgDone] -> Chart/1(PassStBkReclnStgDone)
  If4/2 -> If Action Subsystem7/Action
  If4/1 -> If Action Subsystem8/Action
  If5/2 -> If Action Subsystem27/Action
  If5/1 -> If Action Subsystem28/Action
  Chart/8(PassStFwdBkwdEn) -> If4/1
  Chart/9(PassStBkReclnEn) -> If5/1
  [PassStBkReclnStgDone] -> Logical Operator5/3
  [PassStFwdBkwdStgDone] -> Logical Operator5/4
  Chart/10(R3LCshnFldEn2) -> Terminator_15/1
  Chart/11(R3LCshnFldEn3) -> Terminator_16/1

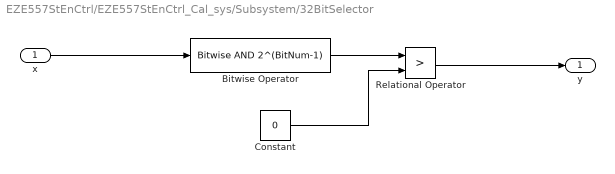
== system EZE557StEnCtrl/EZE557StEnCtrl_Cal_sys/Subsystem/32BitSelector ==
  x : Inport
  Bitwise Operator : simulink/Logic and Bit Operations/Bitwise Operator  logicop=AND  UseBitMask=on  BitMask=2^(BitNum-1)  BitMaskRealWorld=Stored Integer
  Constant : Constant  Value=0  OutDataTypeStr=uint32
  Relational Operator : RelationalOperator  Operator=>  OutDataTypeStr=boolean  RndMeth=Simplest
  y : Outport  VectorParamsAs1DForOutWhenUnconnected=off
  wires:
  Relational Operator/1 -> y/1
  Constant/1 -> Relational Operator/2
  x/1 -> Bitwise Operator/1
  Bitwise Operator/1 -> Relational Operator/1

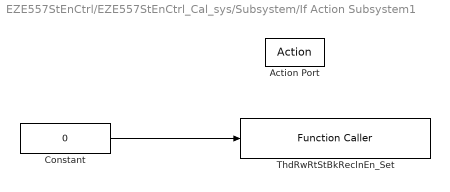
== system EZE557StEnCtrl/EZE557StEnCtrl_Cal_sys/Subsystem/If Action Subsystem1 ==
  Action Port : ActionPort
  Constant : Constant  Value=0  OutDataTypeStr=uint8
  ThdRwRtStBkReclnEn_Set : FunctionCaller  FunctionPrototype=ThdRwRtStBkReclnEn_Set(data)  InputArgumentSpecifications=uint8(1)  OutputArgumentSpecifications=<Enter example>
  wires:
  Constant/1 -> ThdRwRtStBkReclnEn_Set/1

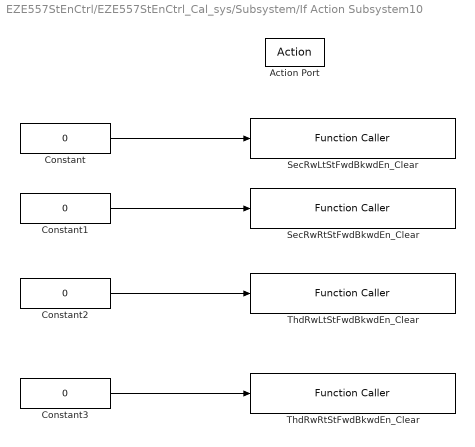
== system EZE557StEnCtrl/EZE557StEnCtrl_Cal_sys/Subsystem/If Action Subsystem10 ==
  Action Port : ActionPort
  Constant{,1..3} (4 alike) : Constant  Value=0  OutDataTypeStr=uint8
  SecRwLtStFwdBkwdEn_Clear : FunctionCaller  FunctionPrototype=SecRwLtStFwdBkwdEn_Clear(data)  InputArgumentSpecifications=uint8(1)  OutputArgumentSpecifications=<Enter example>
  SecRwRtStFwdBkwdEn_Clear : FunctionCaller  FunctionPrototype=SecRwRtStFwdBkwdEn_Clear(data)  InputArgumentSpecifications=uint8(1)  OutputArgumentSpecifications=<Enter example>
  ThdRwLtStFwdBkwdEn_Clear : FunctionCaller  FunctionPrototype=ThdRwLtStFwdBkwdEn_Clear(data)  InputArgumentSpecifications=uint8(1)  OutputArgumentSpecifications=<Enter example>
  ThdRwRtStFwdBkwdEn_Clear : FunctionCaller  FunctionPrototype=ThdRwRtStFwdBkwdEn_Clear(data)  InputArgumentSpecifications=uint8(1)  OutputArgumentSpecifications=<Enter example>
  wires:
  Constant/1 -> SecRwLtStFwdBkwdEn_Clear/1
  Constant1/1 -> SecRwRtStFwdBkwdEn_Clear/1
  Constant2/1 -> ThdRwLtStFwdBkwdEn_Clear/1
  Constant3/1 -> ThdRwRtStFwdBkwdEn_Clear/1

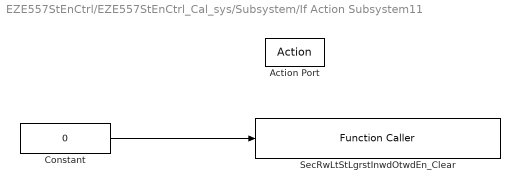
== system EZE557StEnCtrl/EZE557StEnCtrl_Cal_sys/Subsystem/If Action Subsystem11 ==
  Action Port : ActionPort
  Constant : Constant  Value=0  OutDataTypeStr=uint8
  SecRwLtStLgrstInwdOtwdEn_Clear : FunctionCaller  FunctionPrototype=SecRwLtStLgrstInwdOtwdEn_Clear(data)  InputArgumentSpecifications=uint8(1)  OutputArgumentSpecifications=<Enter example>
  wires:
  Constant/1 -> SecRwLtStLgrstInwdOtwdEn_Clear/1

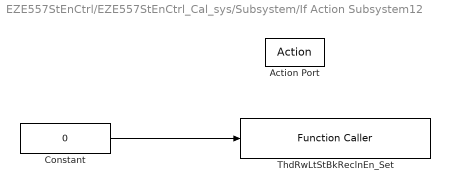
== system EZE557StEnCtrl/EZE557StEnCtrl_Cal_sys/Subsystem/If Action Subsystem12 ==
  Action Port : ActionPort
  Constant : Constant  Value=0  OutDataTypeStr=uint8
  ThdRwLtStBkReclnEn_Set : FunctionCaller  FunctionPrototype=ThdRwLtStBkReclnEn_Set(data)  InputArgumentSpecifications=uint8(1)  OutputArgumentSpecifications=<Enter example>
  wires:
  Constant/1 -> ThdRwLtStBkReclnEn_Set/1

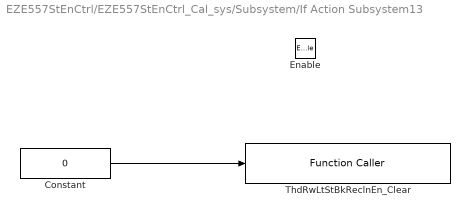
== system EZE557StEnCtrl/EZE557StEnCtrl_Cal_sys/Subsystem/If Action Subsystem13 ==
  Enable : EnablePort
  Constant : Constant  Value=0  OutDataTypeStr=uint8
  ThdRwLtStBkReclnEn_Clear : FunctionCaller  FunctionPrototype=ThdRwLtStBkReclnEn_Clear(data)  InputArgumentSpecifications=uint8(1)  OutputArgumentSpecifications=<Enter example>
  wires:
  Constant/1 -> ThdRwLtStBkReclnEn_Clear/1

== system EZE557StEnCtrl/EZE557StEnCtrl_Cal_sys/Subsystem/If Action Subsystem14 ==
  Action Port : ActionPort
  Constant : Constant  Value=0  OutDataTypeStr=uint8
  SecRwLtStLgrstInwdOtwdEn_Set : FunctionCaller  FunctionPrototype=SecRwLtStLgrstInwdOtwdEn_Set(data)  InputArgumentSpecifications=uint8(1)  OutputArgumentSpecifications=<Enter example>
  wires:
  Constant/1 -> SecRwLtStLgrstInwdOtwdEn_Set/1

== system EZE557StEnCtrl/EZE557StEnCtrl_Cal_sys/Subsystem/If Action Subsystem15 ==
  Action Port : ActionPort
  Constant : Constant  Value=0  OutDataTypeStr=uint8
  SecRwLtStLgrstUpwdDnwdEn_Clear : FunctionCaller  FunctionPrototype=SecRwLtStLgrstUpwdDnwdEn_Clear(data)  InputArgumentSpecifications=uint8(1)  OutputArgumentSpecifications=<Enter example>
  wires:
  Constant/1 -> SecRwLtStLgrstUpwdDnwdEn_Clear/1

== system EZE557StEnCtrl/EZE557StEnCtrl_Cal_sys/Subsystem/If Action Subsystem16 ==
  Action Port : ActionPort
  Constant : Constant  Value=0  OutDataTypeStr=uint8
  SecRwLtStLgrstUpwdDnwdEn_Set : FunctionCaller  FunctionPrototype=SecRwLtStLgrstUpwdDnwdEn_Set(data)  InputArgumentSpecifications=uint8(1)  OutputArgumentSpecifications=<Enter example>
  wires:
  Constant/1 -> SecRwLtStLgrstUpwdDnwdEn_Set/1

== system EZE557StEnCtrl/EZE557StEnCtrl_Cal_sys/Subsystem/If Action Subsystem17 ==
  Action Port : ActionPort
  Constant : Constant  Value=0  OutDataTypeStr=uint8
  ZeroLEn_Clear : FunctionCaller  FunctionPrototype=ZeroLEn_Clear(data)  InputArgumentSpecifications=uint8(1)  OutputArgumentSpecifications=<Enter example>
  wires:
  Constant/1 -> ZeroLEn_Clear/1

== system EZE557StEnCtrl/EZE557StEnCtrl_Cal_sys/Subsystem/If Action Subsystem18 ==
  Action Port : ActionPort
  Constant : Constant  Value=0  OutDataTypeStr=uint8
  ZeroLEn_Set : FunctionCaller  FunctionPrototype=ZeroLEn_Set(data)  InputArgumentSpecifications=uint8(1)  OutputArgumentSpecifications=<Enter example>
  wires:
  Constant/1 -> ZeroLEn_Set/1

== system EZE557StEnCtrl/EZE557StEnCtrl_Cal_sys/Subsystem/If Action Subsystem19 ==
  Action Port : ActionPort
  Constant : Constant  Value=0  OutDataTypeStr=uint8
  SecRwRtStLgrstInwdOtwdEn_Clear : FunctionCaller  FunctionPrototype=SecRwRtStLgrstInwdOtwdEn_Clear(data)  InputArgumentSpecifications=uint8(1)  OutputArgumentSpecifications=<Enter example>
  wires:
  Constant/1 -> SecRwRtStLgrstInwdOtwdEn_Clear/1

== system EZE557StEnCtrl/EZE557StEnCtrl_Cal_sys/Subsystem/If Action Subsystem2 ==
  Enable : EnablePort
  Constant : Constant  Value=0  OutDataTypeStr=uint8
  ThdRwRtStBkReclnEn_Clear : FunctionCaller  FunctionPrototype=ThdRwRtStBkReclnEn_Clear(data)  InputArgumentSpecifications=uint8(1)  OutputArgumentSpecifications=<Enter example>
  wires:
  Constant/1 -> ThdRwRtStBkReclnEn_Clear/1

== system EZE557StEnCtrl/EZE557StEnCtrl_Cal_sys/Subsystem/If Action Subsystem20 ==
  Action Port : ActionPort
  Constant : Constant  Value=0  OutDataTypeStr=uint8
  SecRwRtStLgrstInwdOtwdEn_Set : FunctionCaller  FunctionPrototype=SecRwRtStLgrstInwdOtwdEn_Set(data)  InputArgumentSpecifications=uint8(1)  OutputArgumentSpecifications=<Enter example>
  wires:
  Constant/1 -> SecRwRtStLgrstInwdOtwdEn_Set/1

== system EZE557StEnCtrl/EZE557StEnCtrl_Cal_sys/Subsystem/If Action Subsystem21 ==
  Action Port : ActionPort
  Constant : Constant  Value=0  OutDataTypeStr=uint8
  SecRwRtStLgrstUpwdDnwdEn_Clear : FunctionCaller  FunctionPrototype=SecRwRtStLgrstUpwdDnwdEn_Clear(data)  InputArgumentSpecifications=uint8(1)  OutputArgumentSpecifications=<Enter example>
  wires:
  Constant/1 -> SecRwRtStLgrstUpwdDnwdEn_Clear/1

== system EZE557StEnCtrl/EZE557StEnCtrl_Cal_sys/Subsystem/If Action Subsystem22 ==
  Action Port : ActionPort
  Constant : Constant  Value=0  OutDataTypeStr=uint8
  SecRwRtStLgrstUpwdDnwdEn_Set : FunctionCaller  FunctionPrototype=SecRwRtStLgrstUpwdDnwdEn_Set(data)  InputArgumentSpecifications=uint8(1)  OutputArgumentSpecifications=<Enter example>
  wires:
  Constant/1 -> SecRwRtStLgrstUpwdDnwdEn_Set/1

== system EZE557StEnCtrl/EZE557StEnCtrl_Cal_sys/Subsystem/If Action Subsystem23 ==
  Action Port : ActionPort
  Constant : Constant  Value=0  OutDataTypeStr=uint8
  ZeroREn_Clear : FunctionCaller  FunctionPrototype=ZeroREn_Clear(data)  InputArgumentSpecifications=uint8(1)  OutputArgumentSpecifications=<Enter example>
  wires:
  Constant/1 -> ZeroREn_Clear/1
